simulink model "PVTOL_LMI_AccionIntegral_2024b"  (R2024b)
settings: Solver=ode4  StartTime=0.0  StopTime=100  FixedStep=0.0001  RelTol=1e-3
settings Model: Creator=nestorhernandezcastellanos  LastModifiedBy=nestorhernandezcastellanos
settings ModelReferenceCC: UpdateModelReferenceTargets=IfOutOfDate
settings SFSimCC: SimGPUStackLimitPerThread=51200
settings RTWCC: GPUStackLimitPerThread=51200  GPUComputeCapability=7.5
settings ConfigComp: CovMetricSettings=de  CovBoundaryAbsTol=1.0e-5

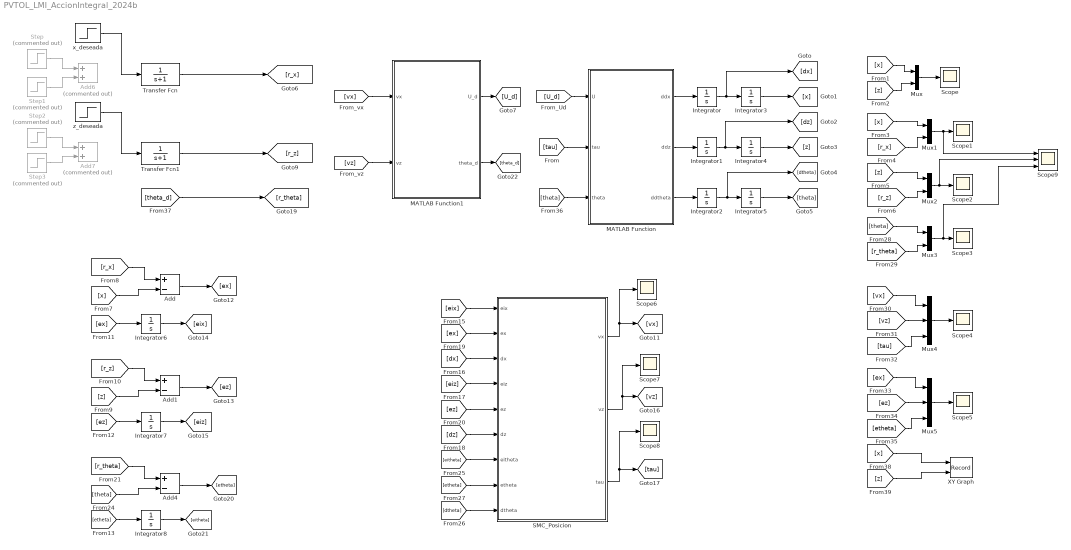
== system PVTOL_LMI_AccionIntegral_2024b ==
  Add : Sum  Inputs=+-
  Add1 : Sum  Inputs=+-
  Add4 : Sum  Inputs=+-
  Add6 : Sum  Commented=on
  Add7 : Sum  Commented=on
  Integrator{,1..8} (9 alike) : Integrator
  MATLAB Function : MATLAB Function  TreatAsAtomicUnit=on
  MATLAB Function1 : MATLAB Function  TreatAsAtomicUnit=on
  Mux{,1..3} (4 alike) : Mux  Inputs=2
  Mux4 : Mux  Inputs=3
  Mux5 : Mux  Inputs=3
  SMC_Posicion : MATLAB Function  TreatAsAtomicUnit=on
  Scope{,1..8} (9 alike) : Scope
  Scope9 : Scope  NumInputPorts=3
  Step : Step  Commented=on  After=3  SampleTime=0
  Step1 : Step  Commented=on  Time=15  After=7  SampleTime=0
  Step2 : Step  Commented=on  After=3  SampleTime=0
  Step3 : Step  Commented=on  Time=15  After=7  SampleTime=0
  Transfer Fcn : TransferFcn  Denominator=[1 1]
  Transfer Fcn1 : TransferFcn  Denominator=[1 1]
  XY Graph : Record  FileSettingsInternal="{\"entries\":[{\"content\":{\"excelSettings\":{\"content\":{},\"type\":\"Streamout.ExcelSettings\"},\"parquetSettings\":{\"content\":{},\"type\":\"Streamout.ParquetSettings\"}},\"type\":\"Streamout.FileSettingStorage\",\"uuid\":\"\"}],\"packageUris\":[\"http:\\/\\/schema.mathworks.com\\/mf0\\/streamout_blocks\\/R2020a\"],\"version\":\"1.0\"}"  Layout=[1 1]  SignalsInternal="{\"entries\":[{\"content\":{\"signals\":[{\"content\":{\"blockPath\":[],\"dimensions\":[1],\"domain\":\"\",\"lineColor\":\"#a2142f\",\"plots\":[ 1 ],\"port\":1,\"signalID\":1,\"signalName\":\"From38\"},\"type\":\"RecordBlkView.Signal\",\"uuid\":\"\"},{\"content\":{\"blockPath\":[],\"dimensions\":[1],\"domain\":\"\",\"lineColor\":\"#139fff\",\"plots\":[ 1 ],\"port\":2,\"signalID\":2,\"signalName\":\"From39\"},\"type\":\"RecordBlkView.Signal\",\"uuid\":\"\"}]},\"type\":\"RecordBlkView.InputSignals\",\"uuid\":\"\"}],\"packageUris\":[\"http:\\/\\/schema.mathworks.com\\/mf0\\/streamout_blocks\\/R2020a\"],\"version\":\"1.0\"}"  VisualizationBindings="{\"xyplotplugin\":{\"info\":[{\"series\":[{\"bindingParametersList\":[{\"parameter\":\"X-Axis\",\"signalID\":1,\"signalName\":\"From38\"},{\"parameter\":\"Y-Axis\",\"signalID\":2,\"signalName\":\"From39\"}],\"seriesID\":0}],\"subplotID\":1}]}}"  CompatibilityTag=XY
  x_deseada : Step  After=5  SampleTime=0
  z_deseada : Step  After=5  SampleTime=0
  wires:
  MATLAB Function/1(ddx) -> Integrator/1
  MATLAB Function/2(ddz) -> Integrator1/1
  MATLAB Function/3(ddtheta) -> Integrator2/1
  Integrator2/1 -> [dtheta], Integrator5/1
  Integrator1/1 -> [dz], Integrator4/1
  Integrator/1 -> [dx], Integrator3/1
  Integrator3/1 -> [x]
  Integrator4/1 -> [z]
  Integrator5/1 -> [theta]
  Mux/1 -> Scope/1
  [z] -> Mux/2
  [x] -> Mux/1
  Transfer Fcn/1 -> [r_x]
  [vx] -> MATLAB Function1/1(vx)
  [vz] -> MATLAB Function1/2(vz)
  [U_d] -> MATLAB Function/1(U)
  MATLAB Function1/1(U_d) -> [U_d]
  [x] -> Mux1/1
  [r_x] -> Mux1/2
  Mux1/1 -> Scope9/1, Scope1/1
  [r_z] -> Mux2/2
  [z] -> Mux2/1
  Transfer Fcn1/1 -> [r_z]
  [tau] -> MATLAB Function/2(tau)
  [r_x] -> Add/1
  [x] -> Add/2
  Add/1 -> [ex]
  Add1/1 -> [ez]
  [z] -> Add1/2
  [r_z] -> Add1/1
  SMC_Posicion/1(vx) -> Scope6/1, [vx]
  SMC_Posicion/2(vz) -> Scope7/1, [vz]
  SMC_Posicion/3(tau) -> Scope8/1, [tau]
  [eix] -> SMC_Posicion/1(eix)
  [theta_d] -> [r_theta]
  [r_theta] -> Add4/1
  [theta] -> Add4/2
  Add4/1 -> [etheta]
  MATLAB Function1/2(theta_d) -> [theta_d]
  [theta] -> Mux3/1
  [r_theta] -> Mux3/2
  Mux4/1 -> Scope4/1
  [vz] -> Mux4/2
  [vx] -> Mux4/1
  [tau] -> Mux4/3
  [etheta] -> Mux5/3
  [ex] -> Mux5/1
  [ez] -> Mux5/2
  Mux5/1 -> Scope5/1
  [theta] -> MATLAB Function/3(theta)
  [x] -> XY Graph/1
  [z] -> XY Graph/2
  Mux2/1 -> Scope2/1, Scope9/2
  Mux3/1 -> Scope3/1, Scope9/3
  Step1/1 -> Add6/2
  Step/1 -> Add6/1
  Step2/1 -> Add7/1
  Step3/1 -> Add7/2
  x_deseada/1 -> Transfer Fcn/1
  z_deseada/1 -> Transfer Fcn1/1
  [ex] -> Integrator6/1
  Integrator6/1 -> [eix]
  Integrator7/1 -> [eiz]
  [ez] -> Integrator7/1
  [etheta] -> Integrator8/1
  Integrator8/1 -> [eitheta]
  [dtheta] -> SMC_Posicion/9(dtheta)
  [etheta] -> SMC_Posicion/8(etheta)
  [eitheta] -> SMC_Posicion/7(eitheta)
  [dz] -> SMC_Posicion/6(dz)
  [ez] -> SMC_Posicion/5(ez)
  [eiz] -> SMC_Posicion/4(eiz)
  [dx] -> SMC_Posicion/3(dx)
  [ex] -> SMC_Posicion/2(ex)

== matlab function PVTOL_LMI_AccionIntegral_2024b/MATLAB Function1 ==
  data: vx input; U_d output; vz input; theta_d output
function [U_d,theta_d] = linealizacion(vx,vz)

g = 9.81;                                  
U_d = sqrt(vx^2 + (vz+g)^2);                 
theta_d = atan2(-vx,vz+g);

== matlab function PVTOL_LMI_AccionIntegral_2024b/MATLAB Function ==
  data: U input; ddx output; tau input; theta input; ddz output; ddtheta output
function [ddx,ddz,ddtheta] = planta(U,tau,theta)

g = 9.81;                                       

ddx = -U*sin(theta);                            
ddz = U*cos(theta)-g;                           
ddtheta = tau;

== matlab function PVTOL_LMI_AccionIntegral_2024b/SMC_Posicion ==
  data: eix input; vx output; vz output; tau output; ex input; dx input; eiz input; ez input; dz input; eitheta input; etheta input; dtheta input
function [vx, vz, tau] = controlador(eix, ex, dx, eiz, ez, dz, eitheta, etheta, dtheta)

% Ganancias
Kx = [4.1622    1.9220   -1.7240];
Kz = [6.7952    3.0067   -3.8919];
Ktau = [34.8889 7.8907 -45.3687];

vx = -Kx*[-ex; dx; eix];
vz = -Kz*[-ez; dz; eiz];
tau = -Ktau*[-etheta; dtheta; eitheta];
